simulink library "lib_AirProps_HeatCapacity"  (R2015a)
settings: Solver=ode45  StartTime=0.0  StopTime=10.0  RelTol=1e-3
settings Model: Creator=jlkratz  LastModifiedBy=jlkratz

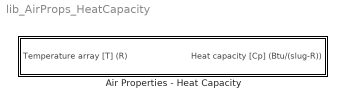
== system lib_AirProps_HeatCapacity ==
  Air Properties - Heat Capacity : Subsystem  mask(TSAT: Air Properties - Heat Capacity Block){BN_M=double(gcb)}
      mask prompts: BN_M "Block name"
      mask help:
      | This function provides an estimate of the heat capacity of air given its temperature. The function uses empirical relations which are valid for dry air in the temperature range of 60K - 2000K (108R - 3600R) and pressures up to 2000MPa. See the block help menu for details. This function is capable of evaluating the heat capacity for various temperatures at the same time given an array of temperature inputs.
      |
      | Units are clearly stated on the inport and outport so assure that your inputs are in the specified units and the output is properly converted to your desired units after the calculation.
      mask Help: web(which('AirProps_TSAT_HeatCapacity.html'),'-helpbrowser')

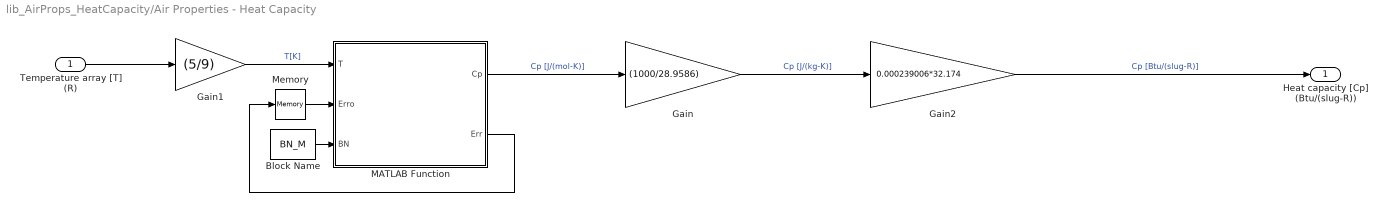
== system lib_AirProps_HeatCapacity/Air Properties - Heat Capacity ==
  Temperature array [T] (R) : Inport
  Block Name : Constant  Value=BN_M
  Gain : Gain  Gain=(1000/28.9586)
  Gain1 : Gain  Gain=(5/9)
  Gain2 : Gain  Gain=0.000239006*32.174
  MATLAB Function : MATLAB Function  TreatAsAtomicUnit=on
  Memory : Memory  X0=zeros(1,2)  InheritSampleTime=on
  Heat capacity [Cp] (Btu/(slug-R)) : Outport
  wires:
  Block Name/1 -> MATLAB Function/3(BN)
  MATLAB Function/2(Err) -> Memory/1
  Memory/1 -> MATLAB Function/2(Erro)
  Gain/1 -> Gain2/1  "Cp [J/(kg-K)]"
  Gain1/1 -> MATLAB Function/1(T)  "T[K]"
  Gain2/1 -> Heat capacity [Cp] (Btu/(slug-R))/1  "Cp [Btu/(slug-R)]"
  Temperature array [T] (R)/1 -> Gain1/1
  MATLAB Function/1(Cp) -> Gain/1  "Cp [J/(mol-K)]"

== matlab function lib_AirProps_HeatCapacity/Air Properties - Heat Capacity/MATLAB Function ==
  data: T input; Cp output; Erro input; BN input; Err output
function [Cp,Err] = HeatCapacity_Air(T,Erro,BN)
%#codegen

%Written By: Jonathan Kratz, NASA GRC
%Date: August 18, 2016
%Descirption: This function calculates the heat capacity of air using
%empirical correlations from:
%   Lemmon, E., Jacobsen, R., Penoncello, S., and Friend, D., 
%   Thermodynamic Properties of Air and Mixtures of Nitrogen, Argon, and 
%   Oxygen From 60 to 2000K at pressure to 2000MPa,” Journal of Physics 
%   Chemistry Reference Data, Vol. 29, No. 3, 2000
%
%Inputs:
%   T - Temperature array of the air in Kelvin (K)
%
%Outputs:
%   Cp - Heat Capacity array corresponding to T in J/(mol-K) 

%Number of element is T to solve for Cp
n = length(T);
Cp = zeros(1,n);

%error checking
Err = Erro;
ErrNum = 1;
if min(T) < 60 && Erro(ErrNum) == 0
    Err(ErrNum) = 1;
    fprintf('warning in %s: At least 1 element of the temperature array is below the temperature range (60-2000K, 108-3600R) which the empirical correlation is valid\n',char(BN));
end
ErrNum = ErrNum + 1;
if max(T) > 2000 && Erro(ErrNum) == 0
    Err(ErrNum) = 1;
    fprintf('warning in %s: At least 1 element of the temperature array is above the temperature range (60-2000K, 108-3600R) which the empirical correlation is valid\n',char(BN));
end

%Coefficients of ideal gas expressions
N = [3.490888032, 2.395525583e-6, 7.172111248e-9, -3.115413101e-13, 0.223806688, 0.791309509, 0.212236768, 0.197938904, 3364.011, 2242.45, 11580.4];

%Gas Constant
R = 8.314510; %universal gas constant J/(mol-K)

for i = 1:n
    %Simplification variables
    u = N(9)/T(i);
    v = N(10)/T(i);
    w = N(11)/T(i);
    %Calculation of Cp (J/mol-K)
    sum = 0;
    for j = 1:4
        sum = sum + N(j)*T(i)^(j-1);
    end
    Cp(i) = R*(sum + N(5)/T(i)^1.5 + (N(6)*u^2.0*exp(u))/(exp(u)-1)^2.0 + (N(7)*v^2.0*exp(v))/((exp(v)-1)^2.0) + ((2.0/3.0)*N(8)*w^2.0*exp(-w))/((2.0/3.0)*exp(-w)+1)^2.0);
end
